simulink model "problem2"  (R2020a)
settings: Solver=VariableStepAuto  StartTime=0.0  StopTime=10.0  RelTol=1e-3
undefined symbols (not defined in the file): b, K1, K2, M1, M2
settings Model: Creator=Riyansh  LastModifiedBy=Riyansh

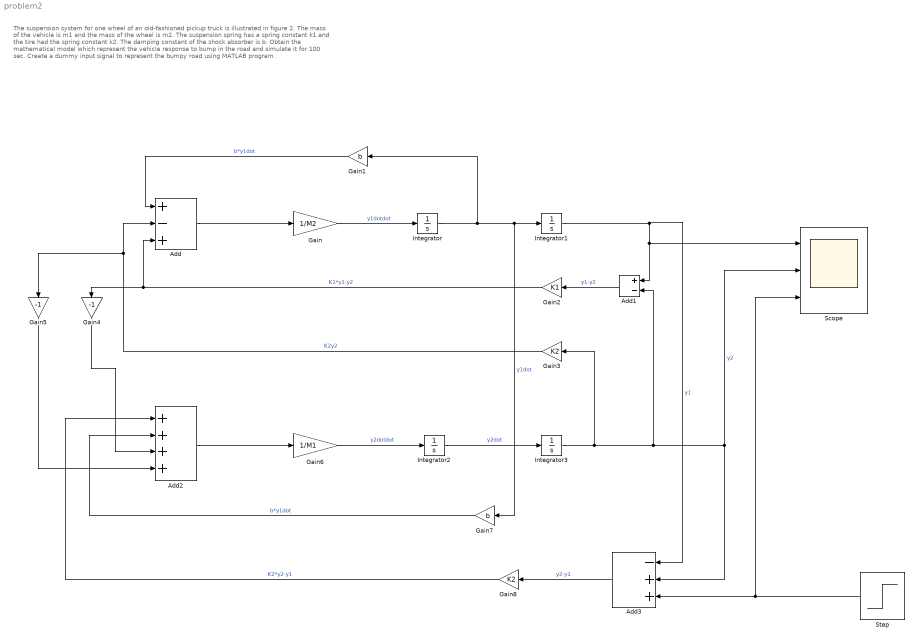
== system problem2 ==
  note: The suspension system for one wheel of an old-fashioned pickup truck is illustrated in figure 2.
      | The mass of the vehicle is m1 and the mass of the wheel is m2. The suspension spring has a spring
      | constant k1 and the tire had the spring constant k2. The damping constant of the shock absorber is b.
      | Obtain the mathematical model which represent the vehicle response to bump in the road and simulate
      | it for 100 sec. Create a dummy input signal to represent the bumpy road using MATLAB program.
  Add : Sum  Inputs=+-+
  Add1 : Sum  Inputs=+-
  Add2 : Sum  Inputs=++++
  Add3 : Sum  Inputs=-++
  Gain : Gain  Gain=1/M2
  Gain1 : Gain  Gain=b
  Gain2 : Gain  Gain=K1
  Gain3 : Gain  Gain=K2
  Gain4 : Gain  Gain=-1
  Gain5 : Gain  Gain=-1
  Gain6 : Gain  Gain=1/M1
  Gain7 : Gain  Gain=b
  Gain8 : Gain  Gain=K2
  Integrator{,1..3} (4 alike) : Integrator
  Scope : Scope  NumInputPorts=3
  Step : Step  SampleTime=0
  wires:
  Gain6/1 -> Integrator2/1  "y2dotdot"
  Gain7/1 -> Add2/2  "b*y1dot"
  Gain3/1 -> Add/2, Gain5/1  "K2y2"
  Integrator1/1 -> Add1/1, Scope/1, Add3/1  "y1"
  Step/1 -> Scope/3, Add3/3
  Add3/1 -> Gain8/1  "y2-y1"
  Gain8/1 -> Add2/1  "K2*y2-y1"
  Gain2/1 -> Add/3, Gain4/1  "K1*y1-y2"
  Integrator3/1 -> Gain3/1, Add1/2, Scope/2, Add3/2  "y2"
  Integrator/1 -> Gain1/1, Gain7/1, Integrator1/1  "y1dot"
  Integrator2/1 -> Integrator3/1  "y2dot"
  Gain5/1 -> Add2/4
  Add1/1 -> Gain2/1  "y1-y2"
  Add/1 -> Gain/1
  Add2/1 -> Gain6/1
  Gain4/1 -> Add2/3
  Gain1/1 -> Add/1  "b*y1dot"
  Gain/1 -> Integrator/1  "y1dotdot"
